simulink model "kkKyocera"  (R2017b)
settings: Solver=ode4  StartTime=0.0  StopTime=1  FixedStep=.001  RelTol=1e-3  EnableMultiTasking=on
values from neighbouring files (symbols this model uses):
  Gcell = insolations(j)    [GenerateVpvInterpolant.m]    (also in Kyocera.m = 1000; Kyoceraupd_interpolant.mat = 1000; QuarterKyocera.m = 1000; commercial_cells_notesandtests.m = Gstring3(i))
  Imax = 1 + currentMargin * Isc * Gcell / 1000    (= 1.05093)    [GenerateVpvInterpolant.m]    (also in Kyocera.m = 9.5; Kyoceraupd_interpolant.mat = 8.371; QuarterKyocera.m = 2.375; idealPVupd_interpolant.mat = 2.09275)
  Ki = 0.0004 * frac    (= 0.0001)    [GenerateVpvInterpolant.m]    (also in Kyocera.m = 0.0004; Kyoceraupd_interpolant.mat = 0.0004; QuarterKyocera.m; idealPVupd_interpolant.mat)
  Kv = -0.0022    [GenerateVpvInterpolant.m]    (also in Kyocera.m; Kyoceraupd_interpolant.mat; QuarterKyocera.m; idealPVupd_interpolant.mat)
  Rseries = 0.0042 * frac    (= 0.00105)    [GenerateVpvInterpolant.m]    (also in Kyocera.m = 0.0042; Kyoceraupd_interpolant.mat = 0.0042; QuarterKyocera.m; idealPVupd_interpolant.mat)
  Rshunt = 91.8 * frac    (= 22.95)    [GenerateVpvInterpolant.m]    (also in Kyocera.m = 91.8; Kyoceraupd_interpolant.mat = 91.8; QuarterKyocera.m; idealPVupd_interpolant.mat)
  Tcell = temperatures(k)    [GenerateVpvInterpolant.m]    (also in Kyocera.m = 25; Kyoceraupd_interpolant.mat = 80; QuarterKyocera.m = 25; commercial_cells_notesandtests.m = Tstring3(i))
libraries: simulink x1
settings Model: Creator=kim800  LastModifiedBy=saeta
settings DataIOCC: LimitDataPoints=on  SaveFormat=Array  SignalLoggingSaveFormat=ModelDataLogs
settings OptimizationCC: ExpressionDepthLimit=2147483647  LifeSpan=inf
settings DebuggingCC: SaveWithParameterizedLinksMsg=none  UnderspecifiedInitializationDetection=Classic  MergeDetectMultiDrivingBlocksExec=none  BlockPriorityViolationMsg=error  MinStepSizeMsg=error  SolverPrmCheckMsg=warning  MultiTaskCondExecSysMsg=none  FcnCallInpInsideContextMsg=warning  SimStateInterfaceChecksumMismatchMsg=error  SFUnexpectedBacktrackingDiag=warning  SFNoUnconditionalDefaultTransitionDiag=warning  SFExecutionAtInitializationDiag=none
settings HardwareCC: ProdBitPerPointer=32  ProdBitPerSizeT=32  ProdBitPerPtrDiffT=32  ProdLargestAtomicFloat=None  ProdIntDivRoundTo=Undefined  ProdEndianess=Unspecified  ProdWordSize=32  ProdHWDeviceType=32-bit Generic
settings ModelReferenceCC: PropagateSignalLabelsOutOfModel=off
settings CodeAppCC: StateflowObjectComments=on
settings GRTTargetCC: TargetLangStandard=C89/C90 (ANSI)  GeneratePreprocessorConditionals=Disable all  CombineOutputUpdateFcns=off  GRTInterface=on
settings ConfigComp: CovMetricSettings=dw  CovHtmlReporting=on  CovSaveCumulativeToWorkspaceVar=on  CovSaveSingleToWorkspaceVar=on  CovExternalEMLEnable=off

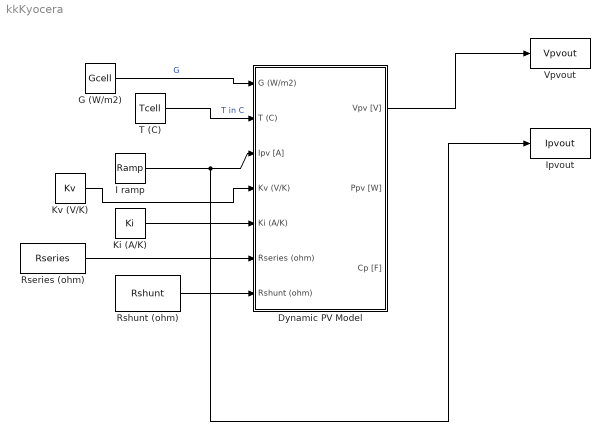
== system kkKyocera ==
  Dynamic PV Model : Subsystem  mask(Photovoltaic String Dynamic Model - Resistances){Iscn=9.26, Vocn=0.6383, Rs=0.0042, Rsh=91.8, Ki=0.004, Kv=-0.001, Ns=1, Vbd=-23.5}
      mask prompts: Iscn "Nominal String Short-Circuit Current (A)"; Vocn "Nominal String Open-Circuit Voltage (V)"; Rs "String Series Resistance [Ohms]"; Rsh "String Shunt Resistance [Ohms]"; Ki "Current Temperature Coefficient (I/K)"; Kv "Voltage Temperature Coefficient (V/K)"; Ns "Number of Cells in Series"; Vbd "Nominal Reverse Breakdown Voltage (V)"
      mask help:
      | Photovoltaic dc model based on string/panel datasheet specifications.
      | Nominal values are based on the string/panel electrical charateristics. Make sure to put the number of cells in the string, otherwise errors may occur.
      | Nominal reverse breakdown voltage:
      | - Should be a negative value.
      | - If not listed on the datasheet, can use -Vmpp*30 as an estimate.
      | - Use 0 to simulate a bypass diode accross the string.
      mask init:
      | % Author: Katherine A. Kim
      | % University of Illinois at Urbana-Champaign
      | % April 2013
      | 
      | % Fit parameters from measured data
      | Ls = 5e-08; %H
      | a = 1.31;
      | % reverse breakdown parameters
      | Isr = 0.0997; %A
      | Kr = 0.0114;
      | % capacitance parameters
      | Cjo = 1.17e-05; %F
      | phio = 0.82; %V
      | tau = 5.76e-06; %s
      | taubd = 0; %s
      | 
      | % Constants
      | k = 1.3806503e-23;   %Boltzmann [J/K]
      | q = 1.60217646e-19;  %Electron charge [C]
      | 
      | % Nominal values
      | Gn = 1000;           %Nominal irradiance [W/m^2] @ 25oC
      | Tn = 25 + 273.15;    %Nominal operating temperature [K]
      | aVtn = a*k*Tn*Ns/q;               %Thermal junction voltage (nominal) 
      | Ion = Iscn/(exp(Vocn/aVtn)-1);    %Nominal diode saturation current
      | Iphn = Iscn;        %Nominal photocurrent approximation
      mask Help:
      | Photovoltaic dc model based on string/panel datasheet specifications.
      | 
      | Nominal values are based on the string/panel electrical charateristics and should be able to be found on the datasheet.
      | 
      | The number of cells in the string/panel is usually listed on the datasheet.
      | 
      | Notes on the nominal reverse breakdown voltage:
      | - Should be a negative value.
      | - If not listed on the datasheet, can use -Vmpp*30 as an estimate.
      | - Use 0 to simulate a bypass diode accross the string.
      | 
      | If errors occur during simulation, check that the number of cells is correct for the voltage ratings.
      | 
      | Example Parameter Values for the E20/435 SOLAR PANEL
      | Nominal String Short-Circuit Current (A)
      | Iscn = 6.43
      | Nominal String Open-Circuit Voltage (V)
      | Vocn = 28.53
      | Nominal String MPP Current (A)
      | Impp = 5.97
      | Nominal String MPP Voltage (V)
      | Vmpp = 24.30
      | Current Temperature Coefficient (I/K)
      | Ki = 3.5-3
      | Voltage Temperature Coefficient (V/K)
      | Kv = -0.0785
      | Number of Cells in Series
      | Ns = 43
      | Nominal Reverse Breakdown Voltage (V)
      | Vbd = -856 or 0 for a bypass diode over the panel
  G (W/m2) : Constant  Value=Gcell
  I ramp : simulink/Sources/Ramp  slope=-Imax  start=0  X0=Imax
  Ipvout : ToWorkspace  VariableName=Ipvout  SampleTime=-1
  Ki (A/K) : Constant  Value=Ki
  Kv (V/K) : Constant  Value=Kv
  Rseries (ohm) : Constant  Value=Rseries
  Rshunt (ohm) : Constant  Value=Rshunt
  T (C) : Constant  Value=Tcell
  Vpvout : ToWorkspace  VariableName=Vpvout  SampleTime=-1
  wires:
  T (C)/1 -> Dynamic PV Model/2(T (C))  "T in C"
  G (W/m2)/1 -> Dynamic PV Model/1(G (W/m2))  "G"
  Dynamic PV Model/1(Vpv [V]) -> Vpvout/1
  I ramp/1 -> Ipvout/1, Dynamic PV Model/3(Ipv [A])
  Kv (V/K)/1 -> Dynamic PV Model/4(Kv (V/K))
  Ki (A/K)/1 -> Dynamic PV Model/5(Ki (A/K))
  Rshunt (ohm)/1 -> Dynamic PV Model/7(Rshunt (ohm))
  Rseries (ohm)/1 -> Dynamic PV Model/6(Rseries (ohm))

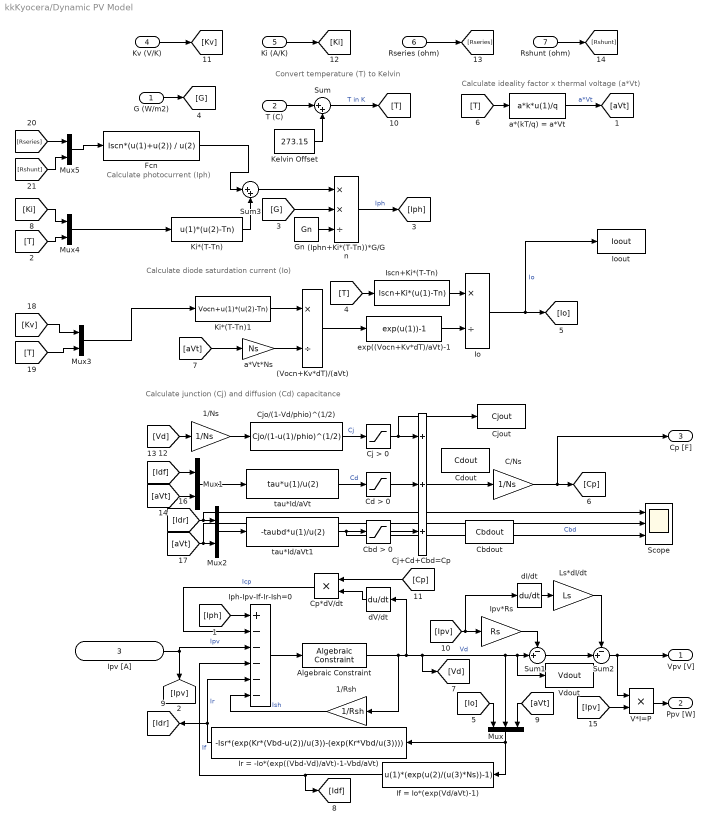
== system kkKyocera/Dynamic PV Model ==
  note: Calculate ideality factor x thermal voltage (a*Vt)
  note: Convert temperature (T) to Kelvin
  note: Calculate diode saturdation current (Io)
  note: Calculate junction (Cj) and diffusion (Cd) capacitance
  note: Calculate photocurrent (Iph)
  G (W/m2) : Inport
  T (C) : Inport  Port=2
  Ipv [A] : Inport  Port=3
  Kv (V/K) : Inport  Port=4
  Ki (A/K) : Inport  Port=5
  Rseries (ohm) : Inport  Port=6
  Rshunt (ohm) : Inport  Port=7
  (Iphn+Ki*(T-Tn))*G/Gn : Product  Inputs=**/
  (Vocn+Kv*dT)/(aVt) : Product  Inputs=*/
  1/Ns : Gain  Gain=1/Ns
  1/Rsh : Gain  Gain=1/Rsh
  Algebraic Constraint : AlgebraicConstraint
  C/Ns : Gain  Gain=1/Ns
  Cbd > 0 : Saturate  UpperLimit=Inf  LowerLimit=0
  Cbdout : ToWorkspace  VariableName=Cbdout  SampleTime=-1
  Cd > 0 : Saturate  UpperLimit=Inf  LowerLimit=0
  Cdout : ToWorkspace  VariableName=Cdout  SampleTime=-1
  Cj > 0 : Saturate  UpperLimit=Inf  LowerLimit=0
  Cj+Cd+Cbd=Cp : Sum  Inputs=+++
  Cjo/(1-Vd/phio)^(1/2) : Fcn  Expr=Cjo/(1-u(1)/phio)^(1/2)
  Cjout : ToWorkspace  VariableName=Cjout  SampleTime=-1
  Cp*dV/dt : Product  Inputs=**
  Fcn : Fcn  Expr=Iscn*(u(1)+u(2)) / u(2)
  Gn : Constant  Value=Gn
  If = Io*(exp(Vd/aVt)-1) : Fcn  Expr=u(1)*(exp(u(2)/(u(3)*Ns))-1)
  Io : Product  Inputs=*/
  Ioout : ToWorkspace  VariableName=Ioout  SampleTime=-1
  Iph-Ipv-If-Ir-Ish=0 : Sum  Inputs=+-----
  Ipv*Rs : Gain  Gain=Rs
  Ir = -Io*(exp((Vbd-Vd)/aVt)-1-Vbd/aVt) : Fcn  Expr=-Isr*(exp(Kr*(Vbd-u(2))/u(3))-(exp(Kr*Vbd/u(3))))
  Iscn+Ki*(T-Tn) : Fcn  Expr=Iscn+Ki*(u(1)-Tn)
  Kelvin Offset : Constant  Value=273.15
  Ki*(T-Tn) : Fcn  Expr=u(1)*(u(2)-Tn)
  Ki*(T-Tn)1 : Fcn  Expr=Vocn+u(1)*(u(2)-Tn)
  Ls*dI/dt : Gain  Gain=Ls
  Mux : Mux  Inputs=3
  Mux{1..5} (5 alike) : Mux  Inputs=2
  Scope : Scope  NumInputPorts=3
  Sum : Sum  Inputs=|++
  Sum1 : Sum  Inputs=-+|
  Sum2 : Sum  Inputs=-+|
  Sum3 : Sum  Inputs=|++
  V*I=P : Product  Inputs=**
  Vdout : ToWorkspace  VariableName=Vdout  SampleTime=-1
  a*(kT/q) = a*Vt : Fcn  Expr=a*k*u(1)/q
  a*Vt*Ns : Gain  Gain=Ns
  dI/dt : Derivative
  dV/dt : Derivative
  exp((Vocn+Kv*dT)/aVt)-1 : Fcn  Expr=exp(u(1))-1
  tau*Id/aVt : Fcn  Expr=tau*u(1)/u(2)
  tau*Id/aVt1 : Fcn  Expr=-taubd*u(1)/u(2)
  Vpv [V] : Outport
  Ppv [W] : Outport  Port=2
  Cp [F] : Outport  Port=3
  wires:
  Kelvin Offset/1 -> Sum/2
  Sum/1 -> [T]  "T in K"
  Sum3/1 -> (Iphn+Ki*(T-Tn))*G/Gn/1
  [G] -> (Iphn+Ki*(T-Tn))*G/Gn/2
  Gn/1 -> (Iphn+Ki*(T-Tn))*G/Gn/3
  (Iphn+Ki*(T-Tn))*G/Gn/1 -> [Iph]  "Iph"
  [aVt] -> a*Vt*Ns/1
  Io/1 -> [Io], Ioout/1  "Io"
  G (W/m2)/1 -> [G]
  T (C)/1 -> Sum/1
  a*(kT/q) = a*Vt/1 -> [aVt]  "a*Vt"
  [T] -> a*(kT/q) = a*Vt/1
  Ki*(T-Tn)/1 -> Sum3/2
  Iscn+Ki*(T-Tn)/1 -> Io/1
  Ki*(T-Tn)1/1 -> (Vocn+Kv*dT)/(aVt)/1
  [T] -> Iscn+Ki*(T-Tn)/1
  exp((Vocn+Kv*dT)/aVt)-1/1 -> Io/2
  (Vocn+Kv*dT)/(aVt)/1 -> exp((Vocn+Kv*dT)/aVt)-1/1
  Ipv [A]/1 -> Iph-Ipv-If-Ir-Ish=0/3, [Ipv]  "Ipv"
  [Iph] -> Iph-Ipv-If-Ir-Ish=0/1
  Iph-Ipv-If-Ir-Ish=0/1 -> Algebraic Constraint/1
  Algebraic Constraint/1 -> dV/dt/1, [Vd], Sum1/2, Vdout/1, Mux/2, 1/Rsh/1  "Vd"
  If = Io*(exp(Vd/aVt)-1)/1 -> [Idf], Iph-Ipv-If-Ir-Ish=0/4  "If"
  Ipv*Rs/1 -> Sum1/1
  [Ipv] -> Ipv*Rs/1, dI/dt/1
  Ls*dI/dt/1 -> Sum2/1
  dI/dt/1 -> Ls*dI/dt/1
  Sum1/1 -> Sum2/2
  Sum2/1 -> V*I=P/1, Vpv [V]/1
  dV/dt/1 -> Cp*dV/dt/2
  Cp*dV/dt/1 -> Iph-Ipv-If-Ir-Ish=0/2  "Icp"
  a*Vt*Ns/1 -> (Vocn+Kv*dT)/(aVt)/2
  [Cp] -> Cp*dV/dt/1
  [Vd] -> 1/Ns/1
  Cj+Cd+Cbd=Cp/1 -> C/Ns/1
  Cjo/(1-Vd/phio)^(1/2)/1 -> Cj > 0/1  "Cj"
  [Idf] -> Mux1/1
  [aVt] -> Mux1/2
  Mux1/1 -> tau*Id/aVt/1
  tau*Id/aVt/1 -> Cd > 0/1  "Cd"
  1/Ns/1 -> Cjo/(1-Vd/phio)^(1/2)/1
  C/Ns/1 -> [Cp], Cp [F]/1
  Cj > 0/1 -> Cj+Cd+Cbd=Cp/1, Cjout/1
  V*I=P/1 -> Ppv [W]/1
  [Ipv] -> V*I=P/2
  1/Rsh/1 -> Iph-Ipv-If-Ir-Ish=0/6  "Ish"
  [Io] -> Mux/1
  [aVt] -> Mux/3
  Mux/1 -> If = Io*(exp(Vd/aVt)-1)/1, Ir = -Io*(exp((Vbd-Vd)/aVt)-1-Vbd/aVt)/1
  Ir = -Io*(exp((Vbd-Vd)/aVt)-1-Vbd/aVt)/1 -> Iph-Ipv-If-Ir-Ish=0/5, [Idr]  "Ir"
  Cd > 0/1 -> Cj+Cd+Cbd=Cp/2
  tau*Id/aVt1/1 -> Cbd > 0/1, Scope/3  "Cbd"
  Cbd > 0/1 -> Cj+Cd+Cbd=Cp/3
  [Idr] -> Mux2/1, Scope/1
  [aVt] -> Mux2/2, Scope/2
  Mux2/1 -> tau*Id/aVt1/1
  Kv (V/K)/1 -> [Kv]
  [Kv] -> Mux3/1
  [T] -> Mux3/2
  Mux3/1 -> Ki*(T-Tn)1/1
  [Ki] -> Mux4/1
  [T] -> Mux4/2
  Mux4/1 -> Ki*(T-Tn)/1
  Ki (A/K)/1 -> [Ki]
  Rseries (ohm)/1 -> [Rseries]
  Rshunt (ohm)/1 -> [Rshunt]
  [Rseries] -> Mux5/1
  [Rshunt] -> Mux5/2
  Mux5/1 -> Fcn/1
  Fcn/1 -> Sum3/1
